simulink model "qsm_sim"  (R2022b)
settings: Solver=ode15s  StartTime=0.0  StopTime=sim_params.t_end  RelTol=1e-4
undefined symbols (not defined in the file or in its folder): environment, init, kite, sim_params, tether, winch
libraries: slpidlib x3
settings Model: Creator=jesse  LastModifiedBy=jesse
settings SolverCC: AlgebraicLoopSolver=TrustRegion
settings DataIOCC: ExternalInput=simIn  SaveState=on
settings DebuggingCC: UnconnectedInputMsg=warning  UnconnectedOutputMsg=warning  UnconnectedLineMsg=warning  SFMachineParentedDataDiag=warning
settings ModelReferenceCC: EnableRefExpFcnMdlSchedulingChecks=on
settings RTWCC: DLArmComputeVersion=19.05

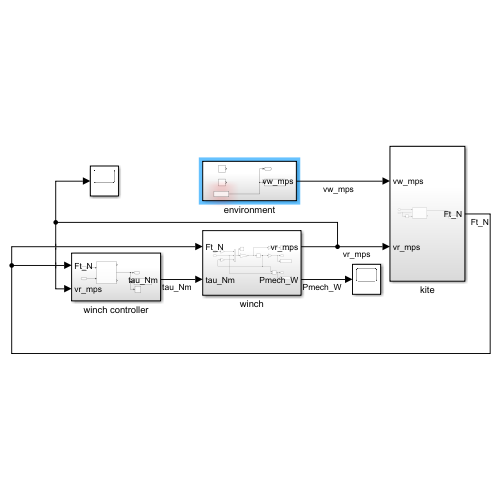
[thumbnail: Simulink's stored preview of the top-level diagram]
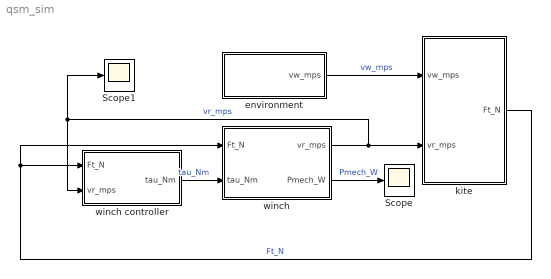
== system qsm_sim ==
  Scope : Scope
  Scope1 : Scope
  environment : Subsystem
  kite : Subsystem
  winch : Subsystem
  winch controller : Subsystem
  wires:
  winch/1(vr_mps) -> Scope1/1, winch controller/2(vr_mps), kite/2(vr_mps)  "vr_mps"
  kite/1(Ft_N) -> winch/1(Ft_N), winch controller/1(Ft_N)  "Ft_N"
  winch controller/1(tau_Nm) -> winch/2(tau_Nm)  "tau_Nm"
  environment/1(vw_mps) -> kite/1(vw_mps)  "vw_mps"
  winch/2(Pmech_W) -> Scope/1  "Pmech_W"

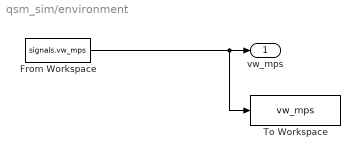
== system qsm_sim/environment ==
  From Workspace : FromWorkspace  VariableName=signals.vw_mps
  To Workspace : ToWorkspace  VariableName=vw_mps  SaveFormat=Timeseries  SampleTime=-1
  vw_mps : Outport
  wires:
  From Workspace/1 -> To Workspace/1, vw_mps/1

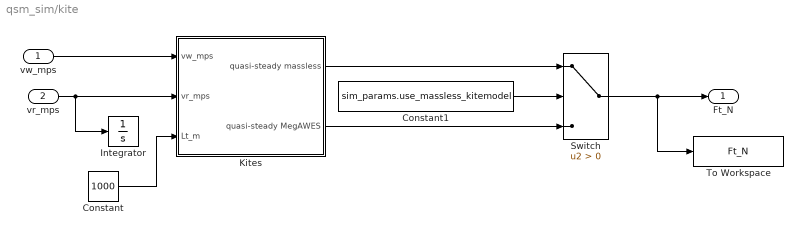
== system qsm_sim/kite ==
  vw_mps : Inport
  vr_mps : Inport  Port=2
  Constant : Constant  Value=1000
  Constant1 : Constant  Value=sim_params.use_massless_kitemodel
  Integrator : Integrator  InitialCondition=init.winch.Lt_m
  Kites : Subsystem
  Switch : Switch  Criteria=u2 > Threshold  SaturateOnIntegerOverflow=off  InputSameDT=off
  To Workspace : ToWorkspace  VariableName=Ft_N  SaveFormat=Timeseries  SampleTime=-1
  Ft_N : Outport
  wires:
  vw_mps/1 -> Kites/1(vw_mps)
  vr_mps/1 -> Integrator/1, Kites/2(vr_mps)
  Switch/1 -> Ft_N/1, To Workspace/1
  Constant/1 -> Kites/3(Lt_m)
  Constant1/1 -> Switch/2
  Kites/2(quasi-steady MegAWES) -> Switch/3
  Kites/1(quasi-steady massless) -> Switch/1

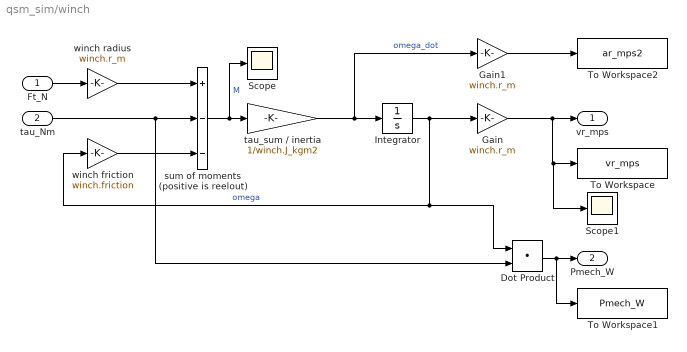
== system qsm_sim/winch ==
  Ft_N : Inport
  tau_Nm : Inport  Port=2
  Dot Product : DotProduct  OutDataTypeStr=Inherit: Inherit via internal rule
  Gain : Gain  Gain=winch.r_m
  Gain1 : Gain  Gain=winch.r_m
  Integrator : Integrator  InitialCondition=init.winch.w_radps;
  Scope : Scope
  Scope1 : Scope
  To Workspace : ToWorkspace  VariableName=vr_mps  SaveFormat=Timeseries  SampleTime=-1
  To Workspace1 : ToWorkspace  VariableName=Pmech_W  SaveFormat=Timeseries  SampleTime=-1
  To Workspace2 : ToWorkspace  VariableName=ar_mps2  SaveFormat=Timeseries  SampleTime=-1
  sum of moments (positive is reelout) : Sum  Inputs=+--
  tau_sum / inertia : Gain  Gain=1/winch.J_kgm2
  winch friction : Gain  Gain=winch.friction
  winch radius : Gain  Gain=winch.r_m
  vr_mps : Outport
  Pmech_W : Outport  Port=2
  wires:
  Ft_N/1 -> winch radius/1
  winch friction/1 -> sum of moments (positive is reelout)/3
  sum of moments (positive is reelout)/1 -> Scope/1, tau_sum / inertia/1  "M"
  Dot Product/1 -> To Workspace1/1, Pmech_W/1
  tau_sum / inertia/1 -> Gain1/1, Integrator/1  "omega_dot"
  tau_Nm/1 -> Dot Product/2, sum of moments (positive is reelout)/2
  winch radius/1 -> sum of moments (positive is reelout)/1
  Integrator/1 -> Gain/1, Dot Product/1, winch friction/1  "omega"
  Gain1/1 -> To Workspace2/1
  Gain/1 -> Scope1/1, To Workspace/1, vr_mps/1

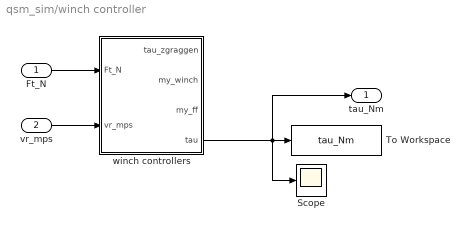
== system qsm_sim/winch controller ==
  Ft_N : Inport
  vr_mps : Inport  Port=2
  Scope : Scope
  To Workspace : ToWorkspace  VariableName=tau_Nm  SaveFormat=Timeseries  SampleTime=-1
  winch controllers : Subsystem
  tau_Nm : Outport
  wires:
  Ft_N/1 -> winch controllers/1(Ft_N)
  vr_mps/1 -> winch controllers/2(vr_mps)
  winch controllers/4(tau) -> tau_Nm/1, Scope/1, To Workspace/1

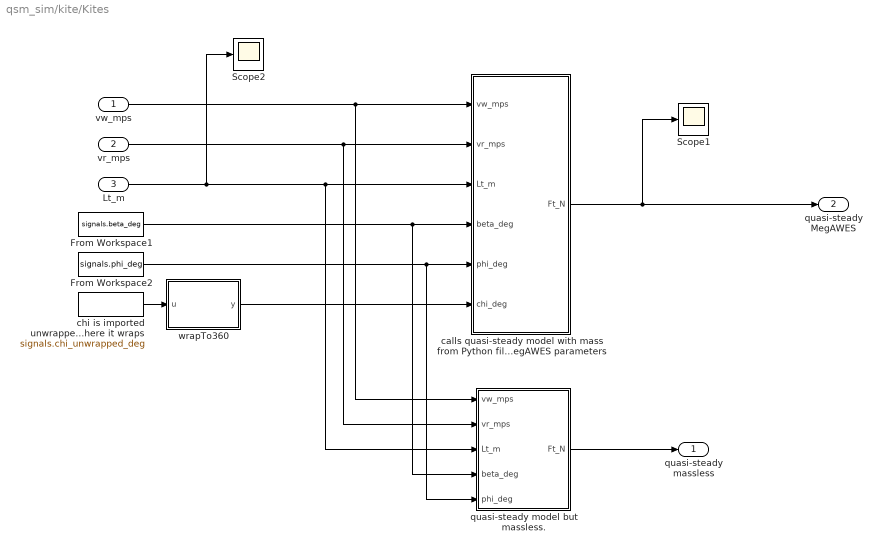
== system qsm_sim/kite/Kites ==
  vw_mps : Inport
  vr_mps : Inport  Port=2
  Lt_m : Inport  Port=3
  From Workspace1 : FromWorkspace  VariableName=signals.beta_deg
  From Workspace2 : FromWorkspace  VariableName=signals.phi_deg
  Scope1 : Scope
  Scope2 : Scope
  calls quasi-steady model with mass from Python file using MegAWES parameters : MATLAB Function  TreatAsAtomicUnit=on
  chi is imported unwrapped so that interpolation doesn't interpolate between the points where it wraps : FromWorkspace  VariableName=signals.chi_unwrapped_deg
  "quasi-steady model but massless. " : MATLAB Function  TreatAsAtomicUnit=on
  wrapTo360 : MATLAB Function  TreatAsAtomicUnit=on
  quasi-steady massless : Outport
  quasi-steady MegAWES : Outport  Port=2
  wires:
  vw_mps/1 -> "quasi-steady model but massless. "/1(vw_mps), calls quasi-steady model with mass from Python file using MegAWES parameters/1(vw_mps)
  Lt_m/1 -> "quasi-steady model but massless. "/3(Lt_m), calls quasi-steady model with mass from Python file using MegAWES parameters/3(Lt_m), Scope2/1
  vr_mps/1 -> "quasi-steady model but massless. "/2(vr_mps), calls quasi-steady model with mass from Python file using MegAWES parameters/2(vr_mps)
  "quasi-steady model but massless. "/1(Ft_N) -> quasi-steady massless/1
  wrapTo360/1(y) -> calls quasi-steady model with mass from Python file using MegAWES parameters/6(chi_deg)
  From Workspace1/1 -> "quasi-steady model but massless. "/4(beta_deg), calls quasi-steady model with mass from Python file using MegAWES parameters/4(beta_deg)
  From Workspace2/1 -> "quasi-steady model but massless. "/5(phi_deg), calls quasi-steady model with mass from Python file using MegAWES parameters/5(phi_deg)
  calls quasi-steady model with mass from Python file using MegAWES parameters/1(Ft_N) -> quasi-steady MegAWES/1, Scope1/1
  chi is imported unwrapped so that interpolation doesn't interpolate between the points where it wraps/1 -> wrapTo360/1(u)

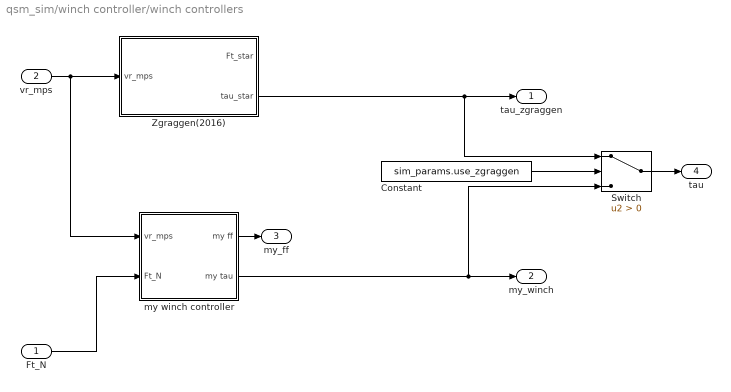
== system qsm_sim/winch controller/winch controllers ==
  Ft_N : Inport
  vr_mps : Inport  Port=2
  Constant : Constant  Value=sim_params.use_zgraggen
  Switch : Switch  Criteria=u2 > Threshold  SaturateOnIntegerOverflow=off  InputSameDT=off
  Zgraggen(2016) : MATLAB Function  TreatAsAtomicUnit=on
  my winch controller : Subsystem
  tau_zgraggen : Outport
  my_winch : Outport  Port=2
  my_ff : Outport  Port=3
  tau : Outport  Port=4
  wires:
  vr_mps/1 -> my winch controller/1(vr_mps), Zgraggen(2016)/1(vr_mps)
  Zgraggen(2016)/2(tau_star) -> Switch/1, tau_zgraggen/1
  Ft_N/1 -> my winch controller/2(Ft_N)
  my winch controller/1(my ff) -> my_ff/1
  my winch controller/2(my tau) -> Switch/3, my_winch/1
  Constant/1 -> Switch/2
  Switch/1 -> tau/1

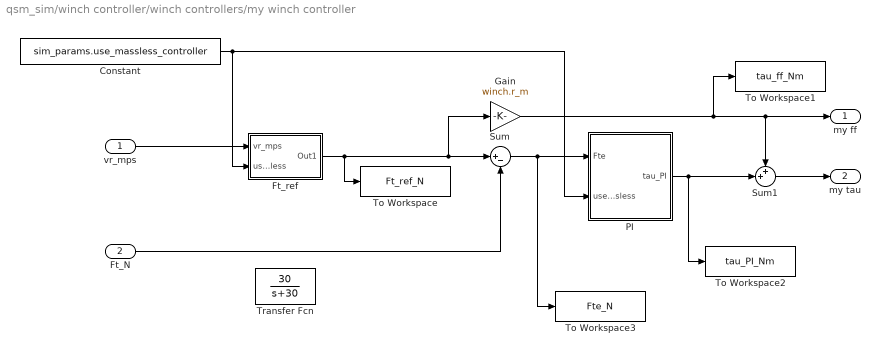
== system qsm_sim/winch controller/winch controllers/my winch controller ==
  vr_mps : Inport
  Ft_N : Inport  Port=2
  Constant : Constant  Value=sim_params.use_massless_controller
  Ft_ref : Subsystem
  Gain : Gain  Gain=winch.r_m
  PI : Subsystem
  Sum : Sum  Inputs=|+-
  Sum1 : Sum  Inputs=++|
  To Workspace : ToWorkspace  VariableName=Ft_ref_N  SaveFormat=Timeseries  SampleTime=-1
  To Workspace1 : ToWorkspace  VariableName=tau_ff_Nm  SaveFormat=Timeseries  SampleTime=-1
  To Workspace2 : ToWorkspace  VariableName=tau_PI_Nm  SaveFormat=Timeseries  SampleTime=-1
  To Workspace3 : ToWorkspace  VariableName=Fte_N  SaveFormat=Timeseries  SampleTime=-1
  Transfer Fcn : TransferFcn  Numerator=[30]  Denominator=[1 30]
  my ff : Outport
  my tau : Outport  Port=2
  wires:
  Sum/1 -> To Workspace3/1, PI/1(Fte)
  Gain/1 -> To Workspace1/1, my ff/1, Sum1/1
  Ft_N/1 -> Sum/2
  Sum1/1 -> my tau/1
  Ft_ref/1(Out1) -> To Workspace/1, Gain/1, Sum/1
  vr_mps/1 -> Ft_ref/1(vr_mps)
  Constant/1 -> Ft_ref/2(use_massless), PI/2(use_massless)
  PI/1(tau_PI) -> Sum1/2, To Workspace2/1

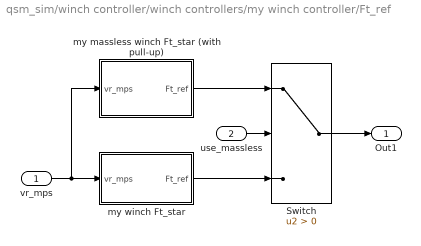
== system qsm_sim/winch controller/winch controllers/my winch controller/Ft_ref ==
  vr_mps : Inport
  use_massless : Inport  Port=2
  Switch : Switch  Criteria=u2 > Threshold  SaturateOnIntegerOverflow=off  InputSameDT=off
  my massless winch Ft_star (with pull-up) : MATLAB Function  TreatAsAtomicUnit=on
  my winch Ft_star : MATLAB Function  TreatAsAtomicUnit=on
  Out1 : Outport
  wires:
  my winch Ft_star/1(Ft_ref) -> Switch/3
  my massless winch Ft_star (with pull-up)/1(Ft_ref) -> Switch/1
  use_massless/1 -> Switch/2
  Switch/1 -> Out1/1
  vr_mps/1 -> my massless winch Ft_star (with pull-up)/1(vr_mps), my winch Ft_star/1(vr_mps)

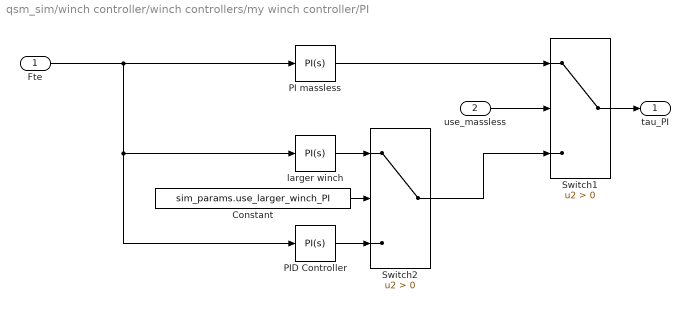
== system qsm_sim/winch controller/winch controllers/my winch controller/PI ==
  Fte : Inport
  use_massless : Inport  Port=2
  Constant : Constant  Value=sim_params.use_larger_winch_PI
  PI massless : slpidlib/PID Controller  Controller=PI  Form=Parallel  TimeDomain=Continuous-time  UseExternalTs=off  SampleTime=0.01  IntegratorMethod=Forward Euler  FilterMethod=Forward Euler  ControllerParametersSource=internal  P=1.481  I=53.53  UseKiTs=off  D=0  N=100  UseFilter=on  TunerSelectOption=Transfer Function Based (PID Tuner App)  InitialConditionSource=internal  InitialConditionForIntegrator=0  InitialConditionForFilter=0  DifferentiatorICPrevScaledInput=0  ExternalReset=none  TrackingMode=off  Kt=1  LimitOutput=off  SatLimitsSource=internal  UpperSaturationLimit=inf  LowerSaturationLimit=-inf  LinearizeAsGain=on  AntiWindupMode=none  Kb=1  LimitIntegrator=off  UpperIntegratorSaturationLimit=inf  LowerIntegratorSaturationLimit=-inf  POutMin=[]  POutMax=[]  IOutMin=[]  IOutMax=[]  DOutMin=[]  DOutMax=[]  NOutMin=[]  NOutMax=[]  SumOutMin=[]  SumOutMax=[]  SaturationOutMin=[]  SaturationOutMax=[]  PParamMin=[]  PParamMax=[]  IParamMin=[]  IParamMax=[]  DParamMin=[]  DParamMax=[]  NParamMin=[]  NParamMax=[]  KbParamMin=[]  KbParamMax=[]  KtParamMin=[]  KtParamMax=[]  KbOutMin=[]  KbOutMax=[]  KtOutMin=[]  KtOutMax=[]  IntegratorOutMin=[]  IntegratorOutMax=[]  FilterOutMin=[]  FilterOutMax=[]  SumI1OutMin=[]  SumI1OutMax=[]  SumI2OutMin=[]  SumI2OutMax=[]  SumI3OutMin=[]  SumI3OutMax=[]  SumI4OutMin=[]  SumI4OutMax=[]  SumDOutMin=[]  SumDOutMax=[]  DifferentiatorOutMin=[]  DifferentiatorOutMax=[]  FilterDiffOutCoefMin=[]  FilterDiffOutCoefMax=[]  ReciprocalOutMin=[]  ReciprocalOutMax=[]  SumDenOutMin=[]  SumDenOutMax=[]  SumNumOutMin=[]  SumNumOutMax=[]  DivideOutMin=[]  DivideOutMax=[]  UdiffTsProdOutMin=[]  UdiffTsProdOutMax=[]  NTsProdOutMin=[]  NTsProdOutMax=[]  UintegralTsProdOutMin=[]  UintegralTsProdOutMax=[]  UngainTsProdOutMin=[]  UngainTsProdOutMax=[]  ClampingZeroOutDataTypeStr=Inherit: Inherit via back propagation  ClampingZeroOutMin=[]  ClampingZeroOutMax=[]  FilterDenConstantOutDataTypeStr=Inherit: Inherit via back propagation  FilterDenConstantOutMin=[]  FilterDenConstantOutMax=[]  PCopyOutDataTypeStr=Inherit: Inherit via back propagation  PCopyOutMin=[]  PCopyOutMax=[]  NCopyOutDataTypeStr=Inherit: Inherit via back propagation  NCopyOutMin=[]  NCopyOutMax=[]  IntegratorContinuousStateAttributes=''  IntegratorStateMustResolveToSignalObject=off  IntegratorRTWStateStorageClass=Auto  FilterContinuousStateAttributes=''  FilterStateMustResolveToSignalObject=off  FilterRTWStateStorageClass=Auto  ParallelPVariant=InternalParameters  IdealPVariant=Disabled  IVariant=InternalParameters  DVariant=Disabled  IntegratorVariant=Continuous  SatVariant=Disabled  AWVariant=Passthrough  PCopyVariant=Disabled  TRVariant=Disabled  FdbkBlocksVariant=Forward  IdealPFdbkVariant=Disabled  SatFdbkVariant=Disabled  DerivativeFilterVariant=Disabled  NVariant=Disabled  NCopyVariant=Disabled_SignalSpec  FilterICVariant=Disabled  IntegratorICVariant=InternalICs  ExternalResetVariant=Disabled  TRSumVariant=Passthrough  SumFdbkVariant=Disabled  SumVariant=Sum_PI  TsampFilterVariant=InternalTs  TsampNgainVariant=Passthrough  TsampIntegralVariant=Passthrough  ExternalSaturationOutDataTypeStr=Inherit: Same as second input
  PID Controller : slpidlib/PID Controller  Controller=PI  Form=Parallel  TimeDomain=Continuous-time  UseExternalTs=off  SampleTime=0.01  IntegratorMethod=Forward Euler  FilterMethod=Forward Euler  ControllerParametersSource=internal  P=0.41768  I=47.9043  UseKiTs=off  D=0  N=100  UseFilter=on  TunerSelectOption=Transfer Function Based (PID Tuner App)  InitialConditionSource=internal  InitialConditionForIntegrator=0  InitialConditionForFilter=0  DifferentiatorICPrevScaledInput=0  ExternalReset=none  TrackingMode=off  Kt=1  LimitOutput=off  SatLimitsSource=internal  UpperSaturationLimit=inf  LowerSaturationLimit=-inf  LinearizeAsGain=on  AntiWindupMode=none  Kb=1  LimitIntegrator=off  UpperIntegratorSaturationLimit=inf  LowerIntegratorSaturationLimit=-inf  POutMin=[]  POutMax=[]  IOutMin=[]  IOutMax=[]  DOutMin=[]  DOutMax=[]  NOutMin=[]  NOutMax=[]  SumOutMin=[]  SumOutMax=[]  SaturationOutMin=[]  SaturationOutMax=[]  PParamMin=[]  PParamMax=[]  IParamMin=[]  IParamMax=[]  DParamMin=[]  DParamMax=[]  NParamMin=[]  NParamMax=[]  KbParamMin=[]  KbParamMax=[]  KtParamMin=[]  KtParamMax=[]  KbOutMin=[]  KbOutMax=[]  KtOutMin=[]  KtOutMax=[]  IntegratorOutMin=[]  IntegratorOutMax=[]  FilterOutMin=[]  FilterOutMax=[]  SumI1OutMin=[]  SumI1OutMax=[]  SumI2OutMin=[]  SumI2OutMax=[]  SumI3OutMin=[]  SumI3OutMax=[]  SumI4OutMin=[]  SumI4OutMax=[]  SumDOutMin=[]  SumDOutMax=[]  DifferentiatorOutMin=[]  DifferentiatorOutMax=[]  FilterDiffOutCoefMin=[]  FilterDiffOutCoefMax=[]  ReciprocalOutMin=[]  ReciprocalOutMax=[]  SumDenOutMin=[]  SumDenOutMax=[]  SumNumOutMin=[]  SumNumOutMax=[]  DivideOutMin=[]  DivideOutMax=[]  UdiffTsProdOutMin=[]  UdiffTsProdOutMax=[]  NTsProdOutMin=[]  NTsProdOutMax=[]  UintegralTsProdOutMin=[]  UintegralTsProdOutMax=[]  UngainTsProdOutMin=[]  UngainTsProdOutMax=[]  ClampingZeroOutDataTypeStr=Inherit: Inherit via back propagation  ClampingZeroOutMin=[]  ClampingZeroOutMax=[]  FilterDenConstantOutDataTypeStr=Inherit: Inherit via back propagation  FilterDenConstantOutMin=[]  FilterDenConstantOutMax=[]  PCopyOutDataTypeStr=Inherit: Inherit via back propagation  PCopyOutMin=[]  PCopyOutMax=[]  NCopyOutDataTypeStr=Inherit: Inherit via back propagation  NCopyOutMin=[]  NCopyOutMax=[]  IntegratorContinuousStateAttributes=''  IntegratorStateMustResolveToSignalObject=off  IntegratorRTWStateStorageClass=Auto  FilterContinuousStateAttributes=''  FilterStateMustResolveToSignalObject=off  FilterRTWStateStorageClass=Auto  ParallelPVariant=InternalParameters  IdealPVariant=Disabled  IVariant=InternalParameters  DVariant=Disabled  IntegratorVariant=Continuous  SatVariant=Disabled  AWVariant=Passthrough  PCopyVariant=Disabled  TRVariant=Disabled  FdbkBlocksVariant=Forward  IdealPFdbkVariant=Disabled  SatFdbkVariant=Disabled  DerivativeFilterVariant=Disabled  NVariant=Disabled  NCopyVariant=Disabled_SignalSpec  FilterICVariant=Disabled  IntegratorICVariant=InternalICs  ExternalResetVariant=Disabled  TRSumVariant=Passthrough  SumFdbkVariant=Disabled  SumVariant=Sum_PI  TsampFilterVariant=InternalTs  TsampNgainVariant=Passthrough  TsampIntegralVariant=Passthrough  ExternalSaturationOutDataTypeStr=Inherit: Same as second input
  Switch1 : Switch  Criteria=u2 > Threshold  SaturateOnIntegerOverflow=off  InputSameDT=off
  Switch2 : Switch  Criteria=u2 > Threshold  SaturateOnIntegerOverflow=off  InputSameDT=off
  larger winch : slpidlib/PID Controller  Controller=PI  Form=Parallel  TimeDomain=Continuous-time  UseExternalTs=off  SampleTime=0.01  IntegratorMethod=Forward Euler  FilterMethod=Forward Euler  ControllerParametersSource=internal  P=67  I=403  UseKiTs=off  D=0  N=100  UseFilter=on  TunerSelectOption=Transfer Function Based (PID Tuner App)  InitialConditionSource=internal  InitialConditionForIntegrator=0  InitialConditionForFilter=0  DifferentiatorICPrevScaledInput=0  ExternalReset=none  TrackingMode=off  Kt=1  LimitOutput=off  SatLimitsSource=internal  UpperSaturationLimit=inf  LowerSaturationLimit=-inf  LinearizeAsGain=on  AntiWindupMode=none  Kb=1  LimitIntegrator=off  UpperIntegratorSaturationLimit=inf  LowerIntegratorSaturationLimit=-inf  POutMin=[]  POutMax=[]  IOutMin=[]  IOutMax=[]  DOutMin=[]  DOutMax=[]  NOutMin=[]  NOutMax=[]  SumOutMin=[]  SumOutMax=[]  SaturationOutMin=[]  SaturationOutMax=[]  PParamMin=[]  PParamMax=[]  IParamMin=[]  IParamMax=[]  DParamMin=[]  DParamMax=[]  NParamMin=[]  NParamMax=[]  KbParamMin=[]  KbParamMax=[]  KtParamMin=[]  KtParamMax=[]  KbOutMin=[]  KbOutMax=[]  KtOutMin=[]  KtOutMax=[]  IntegratorOutMin=[]  IntegratorOutMax=[]  FilterOutMin=[]  FilterOutMax=[]  SumI1OutMin=[]  SumI1OutMax=[]  SumI2OutMin=[]  SumI2OutMax=[]  SumI3OutMin=[]  SumI3OutMax=[]  SumI4OutMin=[]  SumI4OutMax=[]  SumDOutMin=[]  SumDOutMax=[]  DifferentiatorOutMin=[]  DifferentiatorOutMax=[]  FilterDiffOutCoefMin=[]  FilterDiffOutCoefMax=[]  ReciprocalOutMin=[]  ReciprocalOutMax=[]  SumDenOutMin=[]  SumDenOutMax=[]  SumNumOutMin=[]  SumNumOutMax=[]  DivideOutMin=[]  DivideOutMax=[]  UdiffTsProdOutMin=[]  UdiffTsProdOutMax=[]  NTsProdOutMin=[]  NTsProdOutMax=[]  UintegralTsProdOutMin=[]  UintegralTsProdOutMax=[]  UngainTsProdOutMin=[]  UngainTsProdOutMax=[]  ClampingZeroOutDataTypeStr=Inherit: Inherit via back propagation  ClampingZeroOutMin=[]  ClampingZeroOutMax=[]  FilterDenConstantOutDataTypeStr=Inherit: Inherit via back propagation  FilterDenConstantOutMin=[]  FilterDenConstantOutMax=[]  PCopyOutDataTypeStr=Inherit: Inherit via back propagation  PCopyOutMin=[]  PCopyOutMax=[]  NCopyOutDataTypeStr=Inherit: Inherit via back propagation  NCopyOutMin=[]  NCopyOutMax=[]  IntegratorContinuousStateAttributes=''  IntegratorStateMustResolveToSignalObject=off  IntegratorRTWStateStorageClass=Auto  FilterContinuousStateAttributes=''  FilterStateMustResolveToSignalObject=off  FilterRTWStateStorageClass=Auto  ParallelPVariant=InternalParameters  IdealPVariant=Disabled  IVariant=InternalParameters  DVariant=Disabled  IntegratorVariant=Continuous  SatVariant=Disabled  AWVariant=Passthrough  PCopyVariant=Disabled  TRVariant=Disabled  FdbkBlocksVariant=Forward  IdealPFdbkVariant=Disabled  SatFdbkVariant=Disabled  DerivativeFilterVariant=Disabled  NVariant=Disabled  NCopyVariant=Disabled_SignalSpec  FilterICVariant=Disabled  IntegratorICVariant=InternalICs  ExternalResetVariant=Disabled  TRSumVariant=Passthrough  SumFdbkVariant=Disabled  SumVariant=Sum_PI  TsampFilterVariant=InternalTs  TsampNgainVariant=Passthrough  TsampIntegralVariant=Passthrough  ExternalSaturationOutDataTypeStr=Inherit: Same as second input
  tau_PI : Outport
  wires:
  PID Controller/1 -> Switch2/3
  Fte/1 -> larger winch/1, PID Controller/1, PI massless/1
  use_massless/1 -> Switch1/2
  PI massless/1 -> Switch1/1
  Switch1/1 -> tau_PI/1
  larger winch/1 -> Switch2/1
  Switch2/1 -> Switch1/3
  Constant/1 -> Switch2/2

== matlab function qsm_sim/kite/Kites/quasi-steady model but massless.  ==
  data: vw_mps input; Ft_N output; vr_mps input; Lt_m input; beta_deg input; phi_deg input; kite parameter; environment parameter; tether parameter
function Ft_N = fnc(vw_mps, vr_mps, Lt_m, beta_deg, phi_deg, kite, environment, tether)

% Using the massless quasi-steady model from vandervlught2019 using the
% effective lift-to-drag (E) ratio, which takes the tether length into
% account.
% Intermediate results.
q = 0.5 * environment.rho_kgpm3 * vw_mps^2;
E_eff = calc_E_eff(Lt_m, kite, tether);
CR_eff = kite.CL * sqrt(1/E_eff^2 + 1);
f = vr_mps / vw_mps;

% Final result.
Ft_N = q * kite.S_m2 * CR_eff * (1 + E_eff^2) * (cos(beta_deg) * cos(phi_deg) - f)^2;

== matlab function qsm_sim/winch controller/winch controllers/Zgraggen(2016) ==
  data: vr_mps input; Ft_star output; environment parameter; tau_star output; winch parameter; kite parameter; tether parameter
function [Ft_star, tau_star] = fcn(vr_mps, environment, winch, kite, tether)

% Assume a tether length of 1000 m, just like the average condition of my
% winch controller.
Lt_m = 1000;

% From Zgraggen, which is optimal instantaneous power for massless kites
% over beta and phi. So it neglects the retraction phase.
E_eff = calc_E_eff(Lt_m, kite, tether);
CR_eff = kite.CL * sqrt(1/E_eff^2 + 1);
C = 0.5 * environment.rho_kgpm3 * kite.S_m2 * CR_eff * (1 + E_eff^2);

Ft_star = 4 * C * vr_mps^2;
tau_star = Ft_star * winch.r_m;

== matlab function qsm_sim/kite/Kites/calls quasi-steady model with mass from Python file using MegAWES parameters ==
  data: vw_mps input; Ft_N output; vr_mps input; Lt_m input; beta_deg input; phi_deg input; chi_deg input
function Ft_N = fcn(vw_mps, vr_mps, Lt_m, beta_deg, phi_deg, chi_deg)

    % From: https://nl.mathworks.com/matlabcentral/answers/359575-how-to-run-a-python-code-on-simulink
    Ft_N = 0;  % Has to be preassigned, otherwise Simulink throws an error
    coder.extrinsic('py.qsm_wrapper_for_simulink.calc_Ft')  % Python functions have to be run extrinsically, meaning no C code generated
    % TODO: It would be even greater if we could pass it the `kite`,
    % `tether` and `environment` matlab struct.
    out = py.qsm_wrapper_for_simulink.calc_Ft(vw_mps, vr_mps, Lt_m, beta_deg, phi_deg, chi_deg);
    Ft_N = out;
end

== matlab function qsm_sim/winch controller/winch controllers/my winch controller/Ft_ref/my winch Ft_star ==
  data: vr_mps input; Ft_ref output
function Ft_ref  = fcn(vr_mps)

theta = [187486.8, 7784.0, 30865.2];
Ft_star = theta(1) + theta(2) * vr_mps + theta(3) * vr_mps^2;


% Apply minimum tether force if ideal tether force is below it or when
% we're reeling in during the traction phase.
Ft_min = 0.5e6;
Ft_ref = max(Ft_star, Ft_min);
if vr_mps<0
    Ft_ref = Ft_min;
end

== matlab function qsm_sim/kite/Kites/wrapTo360 ==
  data: u input; y output
function y = fcn(u)

y = mod(u, 360);

== matlab function qsm_sim/winch controller/winch controllers/my winch controller/Ft_ref/my massless winch Ft_star (with pull-up) ==
  data: vr_mps input; Ft_ref output; kite parameter; environment parameter; tether parameter
function Ft_ref  = fcn(vr_mps, kite, environment, tether)

% Assume a tether length of 1000 m, just like the average condition of my
% winch controller.
Lt_m = 1000;

% From Zgraggen, which is optimal instantaneous power for massless kites
% over beta and phi. So it neglects the retraction phase.
E_eff = calc_E_eff(Lt_m, kite, tether);
CR_eff = kite.CL * sqrt(1/E_eff^2 + 1);
C = 0.5 * environment.rho_kgpm3 * kite.S_m2 * CR_eff * (1 + E_eff^2);

Ft_star = 4 * C * vr_mps^2;

% The only thing we add to this massless law is the minimum tether force.
Ft_min = 0.5e6;
Ft_ref = max(Ft_star, Ft_min);
if vr_mps<0
    Ft_ref = Ft_min;
end
